simulink model "basic_g_compensation"  (R2021a)
settings: Solver=VariableStepAuto  StartTime=0.0  StopTime=5  RelTol=1e-3
libraries: robotmaniplib x2, robotcorelib x1
settings Model: Creator=ASUS  LastModifiedBy=ASUS

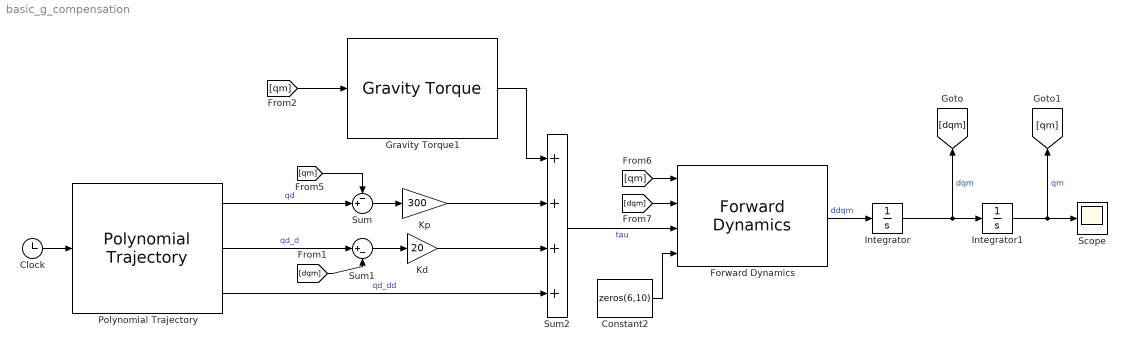
== system basic_g_compensation ==
  Clock : Clock
  Constant2 : Constant  Value=zeros(6,10)
  Forward Dynamics : robotmaniplib/Forward Dynamics  RigidBodyTree=robot  SimulateUsing=Interpreted execution
  Gravity Torque1 : robotmaniplib/Gravity Torque  RigidBodyTree=robot  SimulateUsing=Code generation
  Integrator : Integrator
  Integrator1 : Integrator
  Kd : Gain  Gain=20
  Kp : Gain  Gain=300
  Polynomial Trajectory : robotcorelib/Polynomial Trajectory  WaypointSource=Internal  Waypoints=[ pi/4 pi/4; pi/2 pi/2; pi/8 pi/8; pi/3 pi/3; pi/4 pi/4; pi/5 pi/5]  TimePoints=[ 0, 0.01 ]  TimeInterval=[ 1, 4 ]  Method=Cubic Polynomial  ParameterSource=Internal  VelocityBoundaryCondition=zeros( 6, 2 )  AccelerationBoundaryCondition=zeros( 2, 5 )  SimulateUsing=Interpreted execution
  Scope : Scope
  Sum : Sum  Inputs=-+|
  Sum1 : Sum  Inputs=|+-
  Sum2 : Sum  Inputs=++++
  wires:
  Clock/1 -> Polynomial Trajectory/1
  Polynomial Trajectory/2 -> Sum1/1  "qd_d"
  Forward Dynamics/1 -> Integrator/1  "ddqm"
  Integrator/1 -> [dqm], Integrator1/1  "dqm"
  Sum/1 -> Kp/1
  Sum1/1 -> Kd/1
  Kd/1 -> Sum2/3
  Polynomial Trajectory/3 -> Sum2/4  "qd_dd"
  Constant2/1 -> Forward Dynamics/4
  Sum2/1 -> Forward Dynamics/3  "tau"
  Integrator1/1 -> [qm], Scope/1  "qm"
  [dqm] -> Sum1/2
  Polynomial Trajectory/1 -> Sum/2  "qd"
  [qm] -> Sum/1
  [qm] -> Forward Dynamics/1
  [dqm] -> Forward Dynamics/2
  Kp/1 -> Sum2/2
  Gravity Torque1/1 -> Sum2/1
  [qm] -> Gravity Torque1/1
